simulink model "data_inspector_module"  (R2019a)
settings: Solver=VariableStepAuto  StartTime=0.0  StopTime=inf  RelTol=1e-3
PreLoadFcn:
  | Data_Inspector_Module_setup;
InitFcn:
  | Data_Inspector_Module_setup;
undefined symbols (not defined in the file): AXI4, f_system, Lite
libraries: xbsIndex_r4 x26, simulink x1, dspsigops x1
settings Model: Creator=David Northcote  LastModifiedBy=david

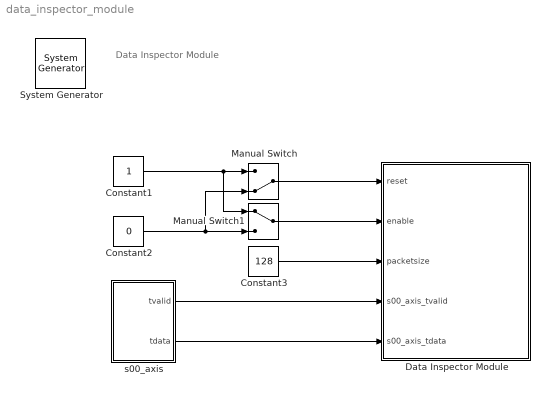
== system data_inspector_module ==
  note: Data Inspector Module
  " System Generator" : xbsIndex_r4/ System Generator  Tag=genX  xilinxfamily=zynquplusRFSOC  part=xczu28dr  speed=-2-e  package=ffvg1517  synthesis_tool=Vivado  clock_wrapper=Clock Enables  directory=./netlist  proj_type=Vivado  Synth_file=Vivado Synthesis Defaults  Impl_file=Vivado Implementation Defaults  testbench=off  simulink_period=1/f_system  sysclk_period=(1/f_system)*1e9  dcm_input_clock_period=10  incr_netlist=off  trim_vbits=Everywhere in SubSystem  dbl_ovrd=According to Block Masks  core_generation=According to Block Masks  run_coregen=off  deprecated_control=off  eval_field=0  block_type=sysgen
  Constant1 : Constant  OutDataTypeStr=boolean  SampleTime=-1
  Constant2 : Constant  Value=0  OutDataTypeStr=boolean  SampleTime=-1
  Constant3 : Constant  Value=128  OutDataTypeStr=uint32  SampleTime=-1
  Data Inspector Module : Subsystem
  Manual Switch : ManualSwitch  CurrentSetting=0
  Manual Switch1 : ManualSwitch
  s00_axis : Subsystem
  wires:
  Constant1/1 -> Manual Switch1/1, Manual Switch/1
  Constant2/1 -> Manual Switch/2, Manual Switch1/2
  Constant3/1 -> Data Inspector Module/3(packetsize)
  Manual Switch/1 -> Data Inspector Module/1(reset)
  s00_axis/1(tvalid) -> Data Inspector Module/4(s00_axis_tvalid)
  s00_axis/2(tdata) -> Data Inspector Module/5(s00_axis_tdata)
  Manual Switch1/1 -> Data Inspector Module/2(enable)

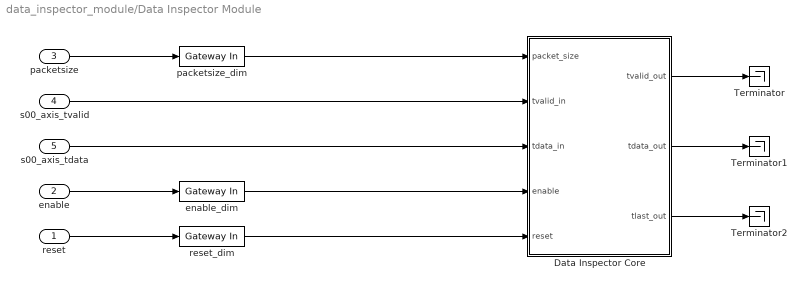
== system data_inspector_module/Data Inspector Module ==
  reset : Inport
  enable : Inport  Port=2
  packetsize : Inport  Port=3
  s00_axis_tvalid : Inport  Port=4
  s00_axis_tdata : Inport  Port=5
  Data Inspector Core : Subsystem
  Terminator : Terminator
  Terminator1 : Terminator
  Terminator2 : Terminator
  enable_dim : xbsIndex_r4/Gateway In  gui_display_data_type=Boolean  arith_type=Boolean  n_bits=32  bin_pt=0  preci_type=Single  exp_width=8  frac_width=24  rows=1  columns=1  quantization="Round  (unbiased: +/- Inf)"  overflow=Saturate  period=1/f_system  UseAsADC=off  ADCChannel='1'  interface=AXI4-Lite  automatic_assignment=off  address_offset=4  intf_name=''  intf_description=''  default_value=0  timing_constraint=None  locs_specified=off  LOCs={}  io_standard={}  inherit_from_input=off  hdl_port=on  dbl_ovrd=off  block_type=gatewayin
  packetsize_dim : xbsIndex_r4/Gateway In  gui_display_data_type=Fixed-point  arith_type=Unsigned  n_bits=32  bin_pt=0  preci_type=Single  exp_width=8  frac_width=24  rows=1  columns=1  quantization="Round  (unbiased: +/- Inf)"  overflow=Saturate  period=1/f_system  UseAsADC=off  ADCChannel='1'  interface=AXI4-Lite  automatic_assignment=off  address_offset=8  intf_name=''  intf_description=''  default_value=0  timing_constraint=None  locs_specified=off  LOCs={}  io_standard={}  inherit_from_input=off  hdl_port=on  dbl_ovrd=off  block_type=gatewayin
  reset_dim : xbsIndex_r4/Gateway In  gui_display_data_type=Boolean  arith_type=Boolean  n_bits=16  bin_pt=14  preci_type=Single  exp_width=8  frac_width=24  rows=1  columns=1  quantization="Round  (unbiased: +/- Inf)"  overflow=Saturate  period=1/f_system  UseAsADC=off  ADCChannel='1'  interface=AXI4-Lite  automatic_assignment=off  address_offset=0  intf_name=''  intf_description=''  default_value=0  timing_constraint=None  locs_specified=off  LOCs={}  io_standard={}  inherit_from_input=off  hdl_port=on  dbl_ovrd=off  block_type=gatewayin
  wires:
  Data Inspector Core/2(tdata_out) -> Terminator1/1
  Data Inspector Core/3(tlast_out) -> Terminator2/1
  reset_dim/1 -> Data Inspector Core/5(reset)
  Data Inspector Core/1(tvalid_out) -> Terminator/1
  reset/1 -> reset_dim/1
  packetsize/1 -> packetsize_dim/1
  s00_axis_tdata/1 -> Data Inspector Core/3(tdata_in)
  packetsize_dim/1 -> Data Inspector Core/1(packet_size)
  s00_axis_tvalid/1 -> Data Inspector Core/2(tvalid_in)
  enable_dim/1 -> Data Inspector Core/4(enable)
  enable/1 -> enable_dim/1

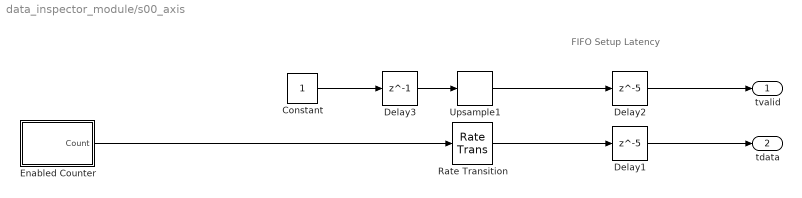
== system data_inspector_module/s00_axis ==
  note: FIFO Setup Latency
  Constant : Constant  OutDataTypeStr=boolean  SampleTime=-1
  Delay1 : Delay  DelayLength=5
  Delay2 : Delay  DelayLength=5
  Delay3 : Delay  DelayLength=1
  Enabled Counter : Subsystem  TreatAsAtomicUnit=on
  Rate Transition : RateTransition  OutPortSampleTime=1/f_system
  Upsample1 : dspsigops/Upsample  N=f_system/(400e3)  phase=0  RateOptions=Allow multirate processing  ic=0  mode=Unused parameter value
  tvalid : Outport
  tdata : Outport  Port=2
  wires:
  Delay2/1 -> tvalid/1
  Delay1/1 -> tdata/1
  Enabled Counter/1(Count) -> Rate Transition/1
  Constant/1 -> Delay3/1
  Rate Transition/1 -> Delay1/1
  Upsample1/1 -> Delay2/1
  Delay3/1 -> Upsample1/1

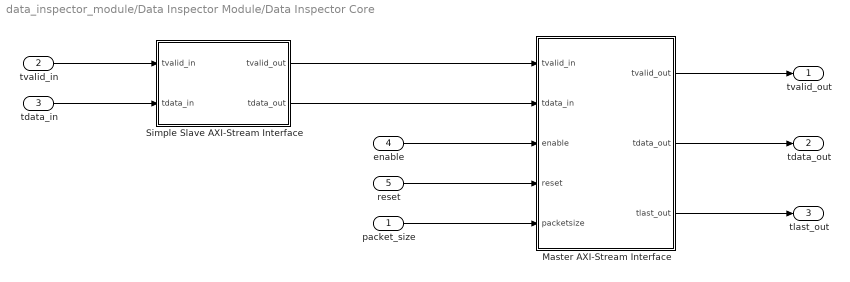
== system data_inspector_module/Data Inspector Module/Data Inspector Core ==
  packet_size : Inport
  tvalid_in : Inport  Port=2
  tdata_in : Inport  Port=3
  enable : Inport  Port=4
  reset : Inport  Port=5
  Master AXI-Stream Interface : Subsystem
  Simple Slave AXI-Stream Interface : Subsystem
  tvalid_out : Outport
  tdata_out : Outport  Port=2
  tlast_out : Outport  Port=3
  wires:
  Master AXI-Stream Interface/2(tdata_out) -> tdata_out/1
  Master AXI-Stream Interface/3(tlast_out) -> tlast_out/1
  Master AXI-Stream Interface/1(tvalid_out) -> tvalid_out/1
  tvalid_in/1 -> Simple Slave AXI-Stream Interface/1(tvalid_in)
  tdata_in/1 -> Simple Slave AXI-Stream Interface/2(tdata_in)
  enable/1 -> Master AXI-Stream Interface/3(enable)
  packet_size/1 -> Master AXI-Stream Interface/5(packetsize)
  Simple Slave AXI-Stream Interface/1(tvalid_out) -> Master AXI-Stream Interface/1(tvalid_in)
  Simple Slave AXI-Stream Interface/2(tdata_out) -> Master AXI-Stream Interface/2(tdata_in)
  reset/1 -> Master AXI-Stream Interface/4(reset)

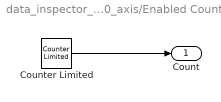
== system data_inspector_module/s00_axis/Enabled Counter ==
  Counter Limited : simulink/Sources/Counter Limited  uplimit=127  tsamp=1/(400e3)
  Count : Outport
  wires:
  Counter Limited/1 -> Count/1

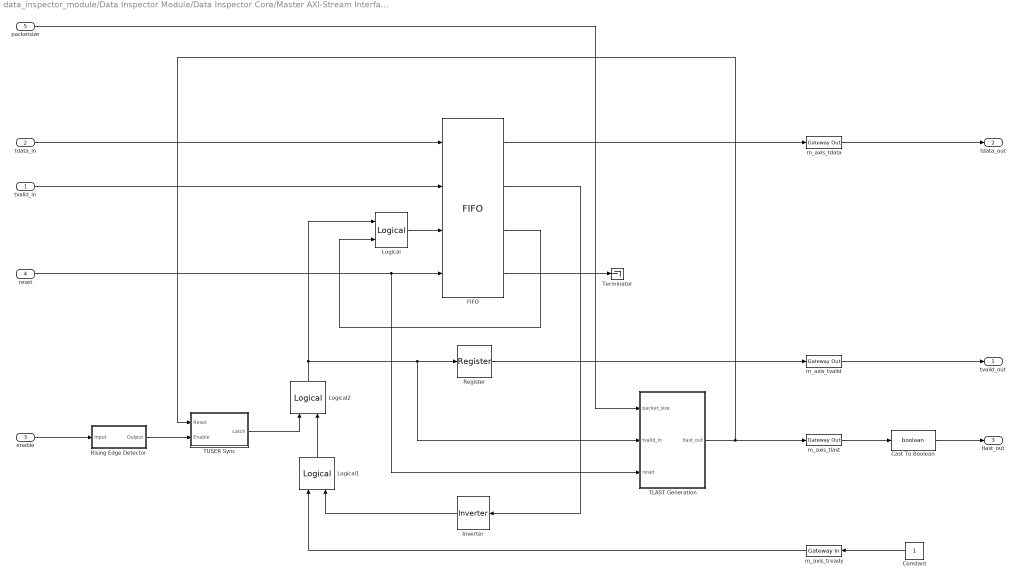
== system data_inspector_module/Data Inspector Module/Data Inspector Core/Master AXI-Stream Interface ==
  tvalid_in : Inport
  tdata_in : Inport  Port=2
  enable : Inport  Port=3
  reset : Inport  Port=4
  packetsize : Inport  Port=5
  Cast To Boolean : DataTypeConversion  OutDataTypeStr=boolean
  Constant : Constant  OutDataTypeStr=boolean  SampleTime=1/f_system
  FIFO : xbsIndex_r4/FIFO  mem_type=Block RAM  performance_options=Standard_FIFO  embedded_registers=off  depth=1K  percent_nbits=1  rst=on  rst_latency=2  en=off  use_dcount=on  use_percent_full_port=off  use_almost_empty=off  almost_empty_thresh=2  use_almost_full=off  use_rd_rst_busy=off  use_wr_rst_busy=off  almost_full_thresh=14  explicit_period=off  dbl_ovrd=off  block_type=fifo
  Inverter : xbsIndex_r4/Inverter  en=off  latency=0  dbl_ovrd=off  block_type=inv
  Logical : xbsIndex_r4/Logical  logical_function=OR  inputs=2  en=off  latency=0  precision=Full  arith_type=Unsigned  n_bits=16  bin_pt=0  align_bp=on  dbl_ovrd=off  block_type=logical
  Logical1 : xbsIndex_r4/Logical  logical_function=AND  inputs=2  en=off  latency=0  precision=Full  arith_type=Unsigned  n_bits=16  bin_pt=0  align_bp=on  dbl_ovrd=off  block_type=logical
  Logical2 : xbsIndex_r4/Logical  logical_function=AND  inputs=2  en=off  latency=0  precision=Full  arith_type=Unsigned  n_bits=16  bin_pt=0  align_bp=on  dbl_ovrd=off  block_type=logical
  Register : xbsIndex_r4/Register  init=0  rst=off  en=off  dbl_ovrd=off  block_type=register
  Rising Edge Detector : Subsystem
  TLAST Generation : Subsystem
  TUSER Sync : Subsystem
  Terminator : Terminator
  m_axis_tdata : xbsIndex_r4/Gateway Out  inherit_from_input=on  hdl_port=on  rows=1  columns=1  UseAsDAC=off  DACChannel='1'  interface=None  automatic_assignment=on  address_offset=hex2dec('00')  intf_name=''  intf_description=''  timing_constraint=None  locs_specified=off  LOCs={}  io_standard={}  block_type=gatewayout
  m_axis_tlast : xbsIndex_r4/Gateway Out  inherit_from_input=on  hdl_port=on  rows=1  columns=1  UseAsDAC=off  DACChannel='1'  interface=None  automatic_assignment=on  address_offset=hex2dec('00')  intf_name=''  intf_description=''  timing_constraint=None  locs_specified=off  LOCs={}  io_standard={}  block_type=gatewayout
  m_axis_tready : xbsIndex_r4/Gateway In  gui_display_data_type=Boolean  arith_type=Boolean  n_bits=16  bin_pt=14  preci_type=Single  exp_width=8  frac_width=24  rows=1  columns=1  quantization="Round  (unbiased: +/- Inf)"  overflow=Saturate  period=1/f_system  UseAsADC=off  ADCChannel='1'  interface=None  automatic_assignment=on  address_offset=hex2dec('00')  intf_name=''  intf_description=''  default_value=0  timing_constraint=None  locs_specified=off  LOCs={}  io_standard={}  inherit_from_input=off  hdl_port=on  dbl_ovrd=off  block_type=gatewayin
  m_axis_tvalid : xbsIndex_r4/Gateway Out  inherit_from_input=on  hdl_port=on  rows=1  columns=1  UseAsDAC=off  DACChannel='1'  interface=None  automatic_assignment=on  address_offset=hex2dec('00')  intf_name=''  intf_description=''  timing_constraint=None  locs_specified=off  LOCs={}  io_standard={}  block_type=gatewayout
  tvalid_out : Outport
  tdata_out : Outport  Port=2
  tlast_out : Outport  Port=3
  wires:
  Constant/1 -> m_axis_tready/1
  m_axis_tdata/1 -> tdata_out/1
  m_axis_tvalid/1 -> tvalid_out/1
  m_axis_tlast/1 -> Cast To Boolean/1
  tvalid_in/1 -> FIFO/2
  reset/1 -> TLAST Generation/3(reset), FIFO/4
  Cast To Boolean/1 -> tlast_out/1
  tdata_in/1 -> FIFO/1
  FIFO/2 -> Inverter/1
  Logical/1 -> FIFO/3
  Inverter/1 -> Logical1/2
  FIFO/3 -> Logical/2
  FIFO/4 -> Terminator/1
  m_axis_tready/1 -> Logical1/1
  FIFO/1 -> m_axis_tdata/1
  TLAST Generation/1(tlast_out) -> TUSER Sync/1(Reset), m_axis_tlast/1
  TUSER Sync/1(Latch) -> Logical2/1
  Logical2/1 -> Logical/1, TLAST Generation/2(tvalid_in), Register/1
  Logical1/1 -> Logical2/2
  Rising Edge Detector/1(Output) -> TUSER Sync/2(Enable)
  enable/1 -> Rising Edge Detector/1(Input)
  packetsize/1 -> TLAST Generation/1(packet_size)
  Register/1 -> m_axis_tvalid/1

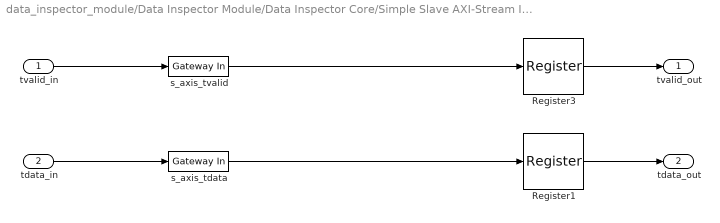
== system data_inspector_module/Data Inspector Module/Data Inspector Core/Simple Slave AXI-Stream Interface ==
  tvalid_in : Inport
  tdata_in : Inport  Port=2
  Register1 : xbsIndex_r4/Register  init=0  rst=off  en=off  dbl_ovrd=off  block_type=register
  Register3 : xbsIndex_r4/Register  init=0  rst=off  en=off  dbl_ovrd=off  block_type=register
  s_axis_tdata : xbsIndex_r4/Gateway In  gui_display_data_type=Fixed-point  arith_type=Unsigned  n_bits=32  bin_pt=0  preci_type=Single  exp_width=8  frac_width=24  rows=1  columns=1  quantization="Round  (unbiased: +/- Inf)"  overflow=Saturate  period=1/f_system  UseAsADC=off  ADCChannel='1'  interface=None  automatic_assignment=on  address_offset=hex2dec('00')  intf_name=''  intf_description=''  default_value=0  timing_constraint=None  locs_specified=off  LOCs={}  io_standard={}  inherit_from_input=off  hdl_port=on  dbl_ovrd=off  block_type=gatewayin
  s_axis_tvalid : xbsIndex_r4/Gateway In  gui_display_data_type=Boolean  arith_type=Boolean  n_bits=16  bin_pt=14  preci_type=Single  exp_width=8  frac_width=24  rows=1  columns=1  quantization="Round  (unbiased: +/- Inf)"  overflow=Saturate  period=1/f_system  UseAsADC=off  ADCChannel='1'  interface=None  automatic_assignment=on  address_offset=hex2dec('00')  intf_name=''  intf_description=''  default_value=0  timing_constraint=None  locs_specified=off  LOCs={}  io_standard={}  inherit_from_input=off  hdl_port=on  dbl_ovrd=off  block_type=gatewayin
  tvalid_out : Outport
  tdata_out : Outport  Port=2
  wires:
  tdata_in/1 -> s_axis_tdata/1
  s_axis_tdata/1 -> Register1/1
  s_axis_tvalid/1 -> Register3/1
  tvalid_in/1 -> s_axis_tvalid/1
  Register3/1 -> tvalid_out/1
  Register1/1 -> tdata_out/1

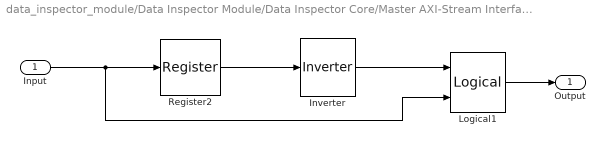
== system data_inspector_module/Data Inspector Module/Data Inspector Core/Master AXI-Stream Interface/Rising Edge Detector ==
  Input : Inport
  Inverter : xbsIndex_r4/Inverter  en=off  latency=0  dbl_ovrd=off  block_type=inv
  Logical1 : xbsIndex_r4/Logical  logical_function=AND  inputs=2  en=off  latency=0  precision=User Defined  arith_type=Boolean  n_bits=16  bin_pt=0  align_bp=on  dbl_ovrd=off  block_type=logical
  Register2 : xbsIndex_r4/Register  init=0  rst=off  en=off  dbl_ovrd=off  block_type=register
  Output : Outport
  wires:
  Register2/1 -> Inverter/1
  Inverter/1 -> Logical1/1
  Logical1/1 -> Output/1
  Input/1 -> Logical1/2, Register2/1

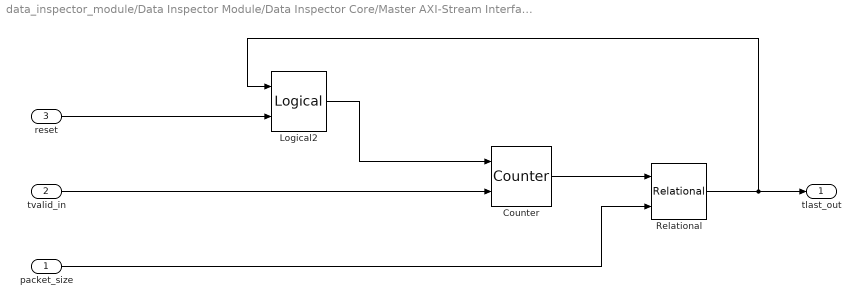
== system data_inspector_module/Data Inspector Module/Data Inspector Core/Master AXI-Stream Interface/TLAST Generation ==
  packet_size : Inport
  tvalid_in : Inport  Port=2
  reset : Inport  Port=3
  Counter : xbsIndex_r4/Counter  cnt_type=Free Running  cnt_to=Inf  operation=Up  start_count=0  cnt_by_val=1  arith_type=Unsigned  n_bits=32  bin_pt=0  load_pin=off  rst=on  en=on  explicit_period=off  period=1  use_behavioral_HDL=off  implementation=Fabric  dbl_ovrd=off  block_type=counter
  Logical2 : xbsIndex_r4/Logical  logical_function=OR  inputs=2  en=off  latency=0  precision=Full  arith_type=Unsigned  n_bits=16  bin_pt=0  align_bp=on  dbl_ovrd=off  block_type=logical
  Relational : xbsIndex_r4/Relational  mode=a>=b  op_type=Bool  en=off  latency=0  dbl_ovrd=off  block_type=relational
  tlast_out : Outport
  wires:
  tvalid_in/1 -> Counter/2
  Logical2/1 -> Counter/1
  reset/1 -> Logical2/2
  Counter/1 -> Relational/1
  packet_size/1 -> Relational/2
  Relational/1 -> tlast_out/1, Logical2/1

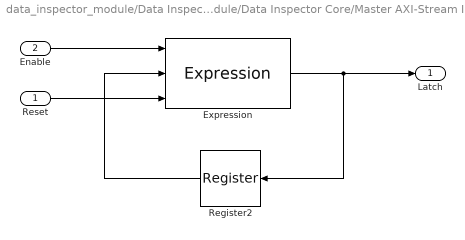
== system data_inspector_module/Data Inspector Module/Data Inspector Core/Master AXI-Stream Interface/TUSER Sync ==
  Reset : Inport
  Enable : Inport  Port=2
  Expression : xbsIndex_r4/Expression  expression=(~R)&((Q^E)|(Q&E))  align_bp=on  en=off  latency=0  precision=Full  arith_type=Unsigned  n_bits=16  bin_pt=0  dbl_ovrd=off  block_type=expr
  Register2 : xbsIndex_r4/Register  init=0  rst=off  en=off  dbl_ovrd=off  block_type=register
  Latch : Outport
  wires:
  Register2/1 -> Expression/2
  Expression/1 -> Latch/1, Register2/1
  Enable/1 -> Expression/1
  Reset/1 -> Expression/3
